simulink model "Main_model"  (R2021b)
settings: Solver=ode23t  StartTime=0.0  StopTime=sim_t_end  RelTol=1e-3
undefined symbols (not defined in the file): ambient_co2, ambient_pressure, ambient_rh, ambient_temp, battery, battery_heat_gen_scale, battery_mass, battery_thermal_mass, cab_air_v_dot, cabin_heater_cmd, cabin_heater_max_power, case_cold_plate_mass, case_cold_plate_thermal_mass, chiller_baffles_n, chiller_tube_length, chiller_tubes_n_rows, compressor_max_m_dot, compressor_ref_m_dot, condenser_air_min_flow_area, condenser_tube_width, const_current, coolant_channel_length, coolant_initial_T, coolant_m_dot, coolant_pipe_cross_sec_area, evaporator_air_cross_sec_area, evaporator_air_min_flow_area, evaporator_tube_width, motor_mc_heat_fraction, n_parallel, power_fraction_rear, ptc_heater_max_power, ptc_heater_thermal_mass, rad_air_v_dot, radiator_air_cross_sec_area, radiator_air_min_flow_area, radiator_tube_width, ref_m_dot, ref_pipe_dia, refrigerant_initial_void_fraction, refrigerant_pipe_cross_sec_area, T_bat_active_cool, T_bat_active_heat, T_bat_passive_cool, T_bat_passive_heat, T_battery_init, T_battery_nom, T_cabin_init, T_cabin_setpoint, T_dcdc_nom, T_DT_high, T_DT_passive_cool, T_DT_whr_active, T_front_gb_nom, T_front_mc_nom, T_front_motor_nom, T_rear_gb_nom, T_rear_mc_nom, T_rear_motor_nom, three_w_valve_max_open_area_factor ... (+3)
libraries: fl_lib x448, nesl_utility x328, SimscapeFluids_lib x134, slpidlib x15, ee_lib x9, simulink x8, LiBatteryElements_lib x4, SignalEditorBlockLib x1
(part 10 of 24)

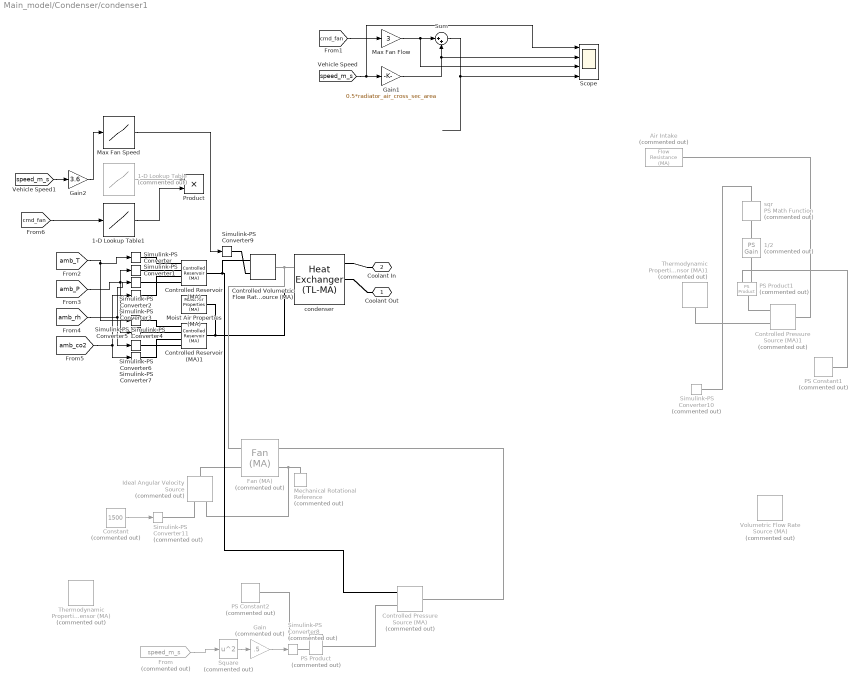
== system Main_model/Condenser/condenser1 ==
  1-D Lookup Table : Lookup_n-D  Commented=on  NumberOfTableDimensions=1  BreakpointsForDimension1=[0, 10, 30, 70, 90,125,161, 180]  Table=[.4462, .4608, .5252, .7346, .8683, 1.2050, 1.5558, 2.15]  InternalRulePriority=Speed  RndMeth=Simplest  InputSameDT=on
  1-D Lookup Table1 : Lookup_n-D  NumberOfTableDimensions=1  BreakpointsForDimension1=[0.5, .75, 1]  Table=[1, 1.15, 1.3]  InternalRulePriority=Speed  RndMeth=Simplest  InputSameDT=on
  1/2 : fl_lib/Physical Signals/Functions/PS Gain  Commented=on  gain=0.5
  Air Intake : fl_lib/Moist Air/Elements/Flow Resistance (MA)  Commented=on  delta_p_nominal=5e-4 MPa  mdot_nominal=1 kg/s  rho_nominal=1.2 kg/m^3  area=.06 m^2  laminar_fraction=1e-3
      settings: SourceProductBaseCode=SS
  Constant : Constant  Commented=on  Value=1500
  Controlled Volumetric Flow Rate Source (MA) : fl_lib/Moist Air/Sources/Controlled Volumetric Flow Rate Source (MA)  power_spec=foundation.enum.power_spec.none  volumetric_flow_conditions=foundation.enum.volumetric_flow_conditions.standard  p_std=0.101325 MPa  T_std=ambient_temp K  RH_std=ambient_rh  area_A=radiator_air_cross_sec_area m^2  area_B=radiator_air_cross_sec_area m^2
      settings: SourceProductBaseCode=SS  InternalSimscapePortConfiguration="{\"Bottom\":[],\"Left\":[{\"id\":\"A\",\"label\":\"A\",\"type\":\"foundation.moist_air.moist_air\"},{\"id\":\"V\",\"label\":\"V\",\"type\":\"input\"}],\"Right\":[{\"id\":\"B\",\"label\":\"B\",\"type\":\"foundation.moist_air.moist_air\"}],\"Top\":[]}"
  Controlled Pressure Source (MA) : fl_lib/Moist Air/Sources/Controlled Pressure Source (MA)  Commented=on  power_spec=foundation.enum.power_spec.none  area_A=0.5*radiator_air_cross_sec_area m^2  area_B=0.5*radiator_air_cross_sec_area m^2
      settings: SourceProductBaseCode=SS  InternalSimscapePortConfiguration="{\"Bottom\":[],\"Left\":[{\"id\":\"A\",\"label\":\"A\",\"type\":\"foundation.moist_air.moist_air\"},{\"id\":\"P\",\"label\":\"P\",\"type\":\"input\"}],\"Right\":[{\"id\":\"B\",\"label\":\"B\",\"type\":\"foundation.moist_air.moist_air\"}],\"Top\":[]}"
  Controlled Pressure Source (MA)1 : fl_lib/Moist Air/Sources/Controlled Pressure Source (MA)  Commented=on  power_spec=foundation.enum.power_spec.isentropic  area_A=.06 m^2  area_B=.06 m^2
      settings: SourceProductBaseCode=SS  InternalSimscapePortConfiguration="{\"Bottom\":[],\"Left\":[{\"id\":\"A\",\"label\":\"A\",\"type\":\"foundation.moist_air.moist_air\"},{\"id\":\"P\",\"label\":\"P\",\"type\":\"input\"}],\"Right\":[{\"id\":\"B\",\"label\":\"B\",\"type\":\"foundation.moist_air.moist_air\"}],\"Top\":[]}"
  Controlled Reservoir (MA) : fl_lib/Moist Air/Elements/Controlled Reservoir (MA)  moisture_spec=foundation.enum.moisture_spec.relative_humidity  trace_gas_spec=foundation.enum.trace_gas_spec.mole_fraction  RH_ws=1  area_A=radiator_air_cross_sec_area m^2  input_error_spec=foundation.enum.input_range_error.warn
      settings: SourceProductBaseCode=SS  InternalSimscapePortConfiguration="{\"Bottom\":[],\"Left\":[{\"id\":\"A\",\"label\":\"A\",\"type\":\"foundation.moist_air.moist_air\"}],\"Right\":[{\"id\":\"T\",\"label\":\"T\",\"type\":\"input\"},{\"id\":\"P\",\"label\":\"P\",\"type\":\"input\"},{\"id\":\"W\",\"label\":\"W\",\"type\":\"input\"},{\"id\":\"G\",\"label\":\"G\",\"type\":\"input\"}],\"Top\":[]}"
  Controlled Reservoir (MA)1 : fl_lib/Moist Air/Elements/Controlled Reservoir (MA)  moisture_spec=foundation.enum.moisture_spec.relative_humidity  trace_gas_spec=foundation.enum.trace_gas_spec.mole_fraction  RH_ws=1  area_A=radiator_air_cross_sec_area m^2  input_error_spec=foundation.enum.input_range_error.warn
      settings: SourceProductBaseCode=SS  InternalSimscapePortConfiguration="{\"Bottom\":[],\"Left\":[{\"id\":\"A\",\"label\":\"A\",\"type\":\"foundation.moist_air.moist_air\"}],\"Right\":[{\"id\":\"T\",\"label\":\"T\",\"type\":\"input\"},{\"id\":\"P\",\"label\":\"P\",\"type\":\"input\"},{\"id\":\"W\",\"label\":\"W\",\"type\":\"input\"},{\"id\":\"G\",\"label\":\"G\",\"type\":\"input\"}],\"Top\":[]}"
  Fan (MA) : SimscapeFluids_lib/Moist Air/Turbomachinery/Fan (MA)  Commented=on  fan_parameterization=fluids.moist_air.turbomachinery.enum.FanParameterization.Nominal  mechanical_power_spec=fluids.moist_air.turbomachinery.enum.FanMechanicalPowerSpec.Power  flow_rate_nominal=1.5 m^3/s  pressure_nominal=300 Pa  eta_nominal=.7  power_nominal=200 W  pressure_max=400 Pa  flow_rate_max=3 m^3/s  omega_ref_nominal=1200 rpm  flow_rate_1D_TLU=[.0278, .0556, .0833, .111, .139, .167] m^3/s  pressure_1D_TLU=[6410, 6375, 6018, 5366, 4501, 3609] Pa  eta_1D_TLU=[.257, .394, .453, .47, .459, .415]  power_1D_TLU=[693, 900, 1107, 1267, 1363, 1452] W  omega_ref_1D=3000 rpm  rho_ref_1D=1.2 kg/m^3  omega_dp_TLU=[2400; 3000; 3600] rpm  flow_rate_dp_TLU=[.0278, .0556, .0833, .111, .139, .167] m^3/s  pressure_dp_TLU=[4111, 4010, 3551, 2881, 2167, 1453; 6410, 6375, 6018, 5366, 4501, 3609; 9217, 9285, 9022, 8428, 7552, 6482] Pa  eta_dp_TLU=[.3, .434, .468, .459, .4, .3; .257, .394, .453, .47, .459, .415; .225, .359, .434, .461, .47, .459]  power_dp_TLU=[381, 514, 632, 697, 753, 809; 693, 900, 1107, 1267, 1363, 1452; 1139, 1438, 1732, 2029, 2233, 2358] W  rho_ref_dp=1.2 kg/m^3  omega_q_TLU=[2990; 3450; 3867] rpm  pressure_q_TLU=[31, 62, 93, 124] Pa  flow_rate_q_TLU=[.802, .759, .703, .611; .936, .902, .862, .81; 1.056, 1.027, .994, .956] m^3/s  eta_q_TLU=[.088, .162, .22, .261; .068, .128, .18, .222; .055, .105, .148, .188]  power_q_TLU=[283, 290, 297, 290; 427, 437, 445, 452; 595, 606, 625, 631] W  rho_ref_q=1.2 kg/m^3  diameter_ratio=1  mech_orientation=fluids.moist_air.turbomachinery.enum.FanMechanicalOrientation.Positive  area_A=0.5*radiator_air_cross_sec_area m^2  area_B=0.5*radiator_air_cross_sec_area m^2
      settings: SourceProductBaseCode=SH  InternalSimscapePortConfiguration="{\"Bottom\":[],\"Left\":[{\"id\":\"A\",\"label\":\"A\",\"type\":\"foundation.moist_air.moist_air\"},{\"id\":\"C\",\"label\":\"C\",\"type\":\"foundation.mechanical.rotational.rotational\"}],\"Right\":[{\"id\":\"B\",\"label\":\"B\",\"type\":\"foundation.moist_air.moist_air\"},{\"id\":\"R\",\"label\":\"R\",\"type\":\"foundation.mechanical.rotational.rotational\"}],\"Top\":[]}"
  From : From  Commented=on  GotoTag=speed_m_s  TagVisibility=global
  Gain : Gain  Commented=on  Gain=.5
  Gain1 : Gain  Gain=0.5*radiator_air_cross_sec_area
  Gain2 : Gain  Gain=3.6
  Ideal Angular Velocity Source : fl_lib/Mechanical/Mechanical Sources/Ideal Angular Velocity Source  Commented=on
  Max Fan Flow : Gain  Gain=3
  Max Fan Speed : Lookup_n-D  NumberOfTableDimensions=1  BreakpointsForDimension1=[0, 10, 30, 70, 90,125,161, 180]  Table=[.76, .78, .81, 1.0, 1.1, 1.36, 1.65, 2.21]  InternalRulePriority=Speed  RndMeth=Simplest  InputSameDT=on
  Mechanical Rotational Reference : fl_lib/Mechanical/Rotational Elements/Mechanical Rotational Reference  Commented=on
  Moist Air Properties (MA) : fl_lib/Moist Air/Utilities/Moist Air Properties (MA)  R_a=287.047 J/(K*kg)  T_TLU=[-56.55, -50 : 10 : -10, -5 : 1 : 5, 10 : 10 : 350]' degC  h_a_TLU=[342.416126230579; 349.005511058471; 359.063577249119; 369.119948684177; 379.175469465129; 389.230944678417; 394.258910928084; 395.264534937366; 396.27017101329; 397.275819932805; 398.281482472874; 399.287159410541; 400.292851523015; 401.298559587728; 402.304284382408; 403.310026685143; 404.315787274435; 409.34489180313; 419.404921755863; 429.468036401264; 439.535033154839; 449.606720928652; 459.683919949603; 469.767460521911; 479.858181001348; 489.956925196484; 500.064539372946; 510.181869006204; 520.309755403634; 530.449032296018; 540.60052248087; 550.765034584465; 560.943359995745; 571.136270013102; 581.344513234296; 591.568813210327; 601.809866375885; 612.068340261954; 622.344871990218; 632.640067043998; 642.95449830646; 653.288705353699; 663.643193987949; 674.018435994423; 684.414869104228; 694.832897145098; 705.272890361557; 715.735185886199; 726.220088344236; 736.727870574087; 747.258774447567; 757.813011774199] kJ/kg  mu_a_TLU=[14.2568883320012; 14.6140127728333; 15.1517277055779; 15.6806860159119; 16.2012351072083; 16.7137043125028; 16.9670071730589; 17.017438062815; 17.0677930842452; 17.1180725309876; 17.1682766951315; 17.2184058672268; 17.2684603362935; 17.3184403898301; 17.3683463138234; 17.4181783927569; 17.4679369096204; 17.7156358640698; 18.2056751785154; 18.68879035749; 19.1652344664982; 19.6352478927873; 20.099059103658; 20.5568853601578; 21.0089333871663; 21.4554000014051; 21.8964726992323; 22.3323302062775; 22.7631429910631; 23.1890737447833; 23.6102778293792; 24.0269036959922; 24.4390932757886; 24.8469823450548; 25.2507008663546; 25.6503733074314; 26.0461189394339; 26.4380521159325; 26.8262825340948; 27.2109154792923; 27.5920520543128; 27.969789394274; 28.3442208682439; 28.7154362685068; 29.0835219883356; 29.4485611890712; 29.8106339572472; 30.1698174524429; 30.5261860464955; 30.8798114546565; 31.2307628592324; 31.5791070262086] s*uPa  k_a_TLU=[19.8808489374933; 20.4162454629695; 21.2248743590758; 22.0232452890903; 22.8117314495857; 23.5906913619588; 23.9767075412237; 24.053639990175; 24.1304826682191; 24.2072359051629; 24.2839000294007; 24.3604753679152; 24.4369622462801; 24.5133609886625; 24.5896719178249; 24.6658953551279; 24.7420316205333; 25.1214164701832; 25.8738283029331; 26.6180150229276; 27.3542674377332; 28.0828634735341; 28.8040686837224; 29.5181367785657; 30.2253101618423; 30.9258204644224; 31.6198890677835; 32.3077276126633; 32.9895384896798; 33.6655153099498; 34.33584335461; 35.0007000027879; 35.6602551380254; 36.3146715334901; 36.9641052165342; 37.6087058133173; 38.248616874307; 38.8839761815308; 39.5149160384798; 40.1415635435708; 40.7640408480637; 41.3824653993118; 41.9969501701893; 42.6076038755117; 43.2145311762238; 43.8178328720941; 44.4176060836121; 45.013944423749; 45.6069381602018; 46.1966743687041; 46.783237077953; 47.3667074066625] mW/(K*m)  p_min=1 kPa  p_max=inf MPa  T_min=-56.55 degC  T_max=350 degC  p_atm=ambient_pressure MPa  T_atm=ambient_temp K  R_w=461.523 J/(K*kg)  p_ws_TLU=[1.71168953425982e-06; 3.93770601979424e-06; 1.28411717710344e-05; 3.80051394873809e-05; .00010323902900209; .000259873810798063; .000401741022116384; .000437454836117844; .000476040820618202; .000517704666185737; .000562664883741207; .000611212677444345; .000657088049117899; .000705987905898279; .000758082381149132; .000813549384183233; .000872574861129522; .00122818386934022; .0023392147667769; .00424668834054807; .00738442748706953; .0123512704340234; .0199458019246787; .0312006356960619; .0474147199263783; .0701823607447713; .10141797792131; .143375967241115; .198665399739302; .270259606559999; .361500961984849; .476101381081492; .618139196722055; .792053183687694; 1.0026345688121; 1.25501792086105; 1.55467186826983; 1.90739066433297; 2.31928772772542; 2.79679245576864; 3.34665187151016; 3.97593907083533; 4.69207105435535; 5.5028394740883; 6.41645928168037; 7.4416425436169; 8.58770832955728; 9.86474556030261; 11.2838558865497; 12.8575218898034; 14.6001810568052; 16.5291642526045] MPa  h_w_vap_TLU=[2836.88241275372; 2837.81392500514; 2838.63937175807; 2838.7309929628; 2838.06905313927; 2836.62597341095; 2835.60023952573; 2835.37006381376; 2835.13143158077; 2834.88429145066; 2834.62859062897; 2500.93420564316; 2498.55329907119; 2496.17495082036; 2493.79885912205; 2491.42474723191; 2489.05236104642; 2477.20875029194; 2453.54955988604; 2429.83856603313; 2406.00136954922; 2381.97406342174; 2357.69101156389; 2333.08088387814; 2308.06565480412; 2282.56034405021; 2256.47287422313; 2229.70428017508; 2202.14968030993; 2173.69998896199; 2144.24368406447; 2113.66758247452; 2081.85585110571; 2048.68725710494; 2014.03141249899; 1977.7449923284; 1939.66849592886; 1899.62342931686; 1857.40930169838; 1812.79975416601; 1765.53721731251; 1715.32525772152; 1661.81700477787; 1604.59703745016; 1543.1534616334; 1476.83692476464; 1404.80240352424; 1325.92091736114; 1238.61667822208; 1140.5102987018; 1027.62017777647; 892.733785613825] kJ/kg  h_w_TLU=[2396.55944251649; 2408.68643343608; 2427.1988031141; 2445.702165897; 2464.18429108356; 2482.62529466839; 2491.82135326629; 2493.6580151792; 2495.49372578218; 2497.32843835745; 2499.16210446923; 2500.99462758899; 2502.83092214066; 2504.6665223621; 2506.50140563013; 2508.335548891; 2510.16892865793; 2519.32352241995; 2537.56068088674; 2555.67742615292; 2573.6403223998; 2591.4109179101; 2608.9455037701; 2626.19492016262; 2643.10444358428; 2659.61377634497; 2675.58278696023; 2696.1846256545; 2716.49989553741; 2736.6235210957; 2756.61216047011; 2776.50561773853; 2796.33378922508; 2816.11979583049; 2835.88181423877; 2855.63430574511; 2875.38889327595; 2895.15500577172; 2914.94035964689; 2934.75132290228; 2954.59319330244; 2974.47041285505; 2994.38673458964; 3014.34535328009; 3034.34900867103; 3054.40006755764; 3074.50058946898; 3094.65237953784; 3114.85703128106; 3135.11596137801; 3155.43043805905; 3175.80160435813] kJ/kg  mu_w_TLU=[6.81365662228272; 7.04953750742707; 7.40970098298307; 7.76991278093907; 8.13017290129507; 8.49048134405107; 8.67065368632907; 8.70668960445667; 8.74272600580827; 8.77876289038387; 8.81480025818347; 8.85083810920707; 8.88687644345467; 8.92291526092627; 8.95895456162187; 8.99499434554147; 9.03103461268507; 9.21124319676307; 9.57169660671907; 9.93219833907507; 10.2927483938311; 10.6533467709871; 11.0139934705431; 11.3746884924991; 11.7354318368551; 12.0962235036111; 12.4570634927671; 12.8179518043231; 13.1788884382791; 13.5398733946351; 13.9009066733911; 14.2619882745471; 14.6231181981031; 14.9842964440591; 15.3455230124151; 15.7067979031711; 16.0681211163271; 16.4294926518831; 16.7909125098391; 17.1523806901951; 17.5138971929511; 17.8754620181071; 18.2370751656631; 18.5987366356191; 18.9604464279751; 19.3222045427311; 19.6840109798871; 20.0458657394431; 20.4077688213991; 20.7697202257551; 21.1317199525111; 21.4937680016671] s*uPa  k_w_TLU=[11.46288215976; 11.941997488935; 12.676358586935; 13.414208884935; 14.155548382935; 14.900377080935; 15.274099879935; 15.348949115735; 15.423833243535; 15.498752263335; 15.573706175135; 15.648694978935; 15.723718674735; 15.798777262535; 15.873870742335; 15.948999114135; 16.024162377935; 16.400502076935; 17.155798374935; 17.914583872935; 18.676858570935; 19.442622468935; 20.211875566935; 20.984617864935; 21.760849362935; 22.540570060935; 23.323779958935; 24.110479056935; 24.900667354935; 25.694344852935; 26.491511550935; 27.292167448935; 28.096312546935; 28.903946844935; 29.715070342935; 30.529683040935; 31.347784938935; 32.169376036935; 32.994456334935; 33.823025832935; 34.655084530935; 35.490632428935; 36.329669526935; 37.172195824935; 38.018211322935; 38.867716020935; 39.720709918935; 40.577193016935; 41.437165314935; 42.300626812935; 43.167577510935; 44.038017408935] mW/(K*m)  D_w=25 mm^2/s  trace_gas_model=foundation.enum.trace_gas_model.none  R_g=188.923 J/(K*kg)  h_g_TLU=[439.555216260064; 444.670268200251; 452.538618847003; 460.487124258496; 468.522588768941; 476.649415958793; 480.74798538725; 481.57054318762; 482.394052398751; 483.218514288831; 484.043930029015; 484.870300696555; 485.697627277859; 486.525910671489; 487.355151691079; 488.185351068185; 489.016509455051; 493.186704139431; 501.599194953048; 510.107689961685; 518.711611080182; 527.410026793075; 536.201764778798; 545.085474203452; 554.059675505208; 563.122805485367; 572.27325096919; 581.509373027928; 590.829525105886; 600.232066705818; 609.715373581392; 619.277845178105; 628.917909922924; 638.634028838794; 648.424697859328; 658.288449140109; 668.223851601449; 678.229510889093; 688.304068901113; 698.44620299875; 708.654624994591; 718.928079991818; 729.265345132425; 739.665228299475; 750.126566808087; 760.648226111439; 771.229098541268; 781.868102096908; 792.564179292476; 803.316296068366; 814.123440770426; 824.984623198037] kJ/kg  mu_g_TLU=[10.8921054191698; 11.2215357085649; 11.7233300740382; 12.2234238147811; 12.7215124453467; 13.2173328890673; 13.4643203184773; 13.5136406274989; 13.562934752385; 13.6122025024997; 13.6614436900741; 13.7106581301692; 13.7598456406398; 13.8090060420983; 13.8581391578796; 13.9072448140062; 13.9563228391538; 14.2012926853717; 14.6890687376044; 15.1738428124161; 15.6554929043332; 16.1339159800463; 16.6090257998657; 17.0807510097148; 17.5490334645512; 18.0138267508952; 18.4750948814453; 18.9328111390399; 19.3869570507278; 19.8375214755778; 20.2844997922255; 20.7278931741254; 21.1677079421287; 21.6039549853963; 22.036649242835; 22.4658092382469; 22.8914566632375; 23.3136160026627; 23.7323141980278; 24.1475803447965; 24.5594454200432; 24.9679420372927; 25.3731042257492; 25.774967231431; 26.1735673380029; 26.5689417053362; 26.9611282240413; 27.350165384404; 27.73609215832; 28.118947892972; 28.4987722151178; 28.8756049449796] s*uPa  k_g_TLU=[10.489430678843; 10.9507672150864; 11.666197960308; 12.392559739764; 13.1299519771612; 13.8778409888416; 14.2554325416312; 14.3312274189707; 14.4071122346908; 14.4830860227061; 14.5591478179508; 14.6352966574703; 14.7115315815553; 14.787851634907; 14.8642558678259; 14.9407433374142; 15.0173131087819; 15.401364480906; 16.1751373988038; 16.9558134611595; 17.7432208682398; 18.5366976599676; 19.3360988502003; 20.1412225692689; 20.9517507672929; 21.7672310558863; 22.5871115634685; 23.4107980865695; 24.2377021890869; 25.0672663781241; 25.8989689893876; 26.732318357514; 27.5668446164644; 28.4020933015927; 29.2376215872816; 30.0729965057542; 30.9077942826816; 31.7416001931033; 32.5740086297993; 33.4046232539953; 34.2330571812868; 35.0589331874899; 35.8818839295189; 36.701552179391; 37.5175910702657; 38.3296643536716; 39.1374466671854; 39.9406238119064; 40.7388930391313; 41.5319633456945; 42.3195557774861; 43.1014037407076] mW/(K*m)  D_g=16 mm^2/s
      settings: SourceProductBaseCode=SS
  PS Constant1 : fl_lib/Physical Signals/Sources/PS Constant  Commented=on  constant=1.2 kg/m^3
  PS Constant2 : fl_lib/Physical Signals/Sources/PS Constant  Commented=on  constant=1.2 kg/m^3
  PS Product : fl_lib/Physical Signals/Functions/PS Product  Commented=on
  PS Product1 : fl_lib/Physical Signals/Functions/PS Product  Commented=on
  Product : Product
  Scope : Scope  NumInputPorts=4
  Simulink-PS Converter : nesl_utility/Simulink-PS Converter  PhysicalDomain=network_engine_domain  SubClassName=ps_input  LeftPortType=input  RightPortType=output  PseudoPeriodic=off  Frequencies=[]  NoiseDistribution=none  NoiseParameters=[]  Unit=K  AffineConversion=off  FilteringAndDerivatives=provide  SimscapeFilterOrder=1  InputFilterTimeConstant=0.001  UdotUserProvided=0
      settings: SourceProductBaseCode=PW,SS
  Simulink-PS Converter1 : nesl_utility/Simulink-PS Converter  PhysicalDomain=network_engine_domain  SubClassName=ps_input  LeftPortType=input  RightPortType=output  PseudoPeriodic=off  Frequencies=[]  NoiseDistribution=none  NoiseParameters=[]  Unit=MPa  AffineConversion=off  FilteringAndDerivatives=provide  SimscapeFilterOrder=1  InputFilterTimeConstant=0.001  UdotUserProvided=0
      settings: SourceProductBaseCode=PW,SS
  Simulink-PS Converter10 : nesl_utility/Simulink-PS Converter  Commented=on  PhysicalDomain=network_engine_domain  SubClassName=ps_input  LeftPortType=input  RightPortType=output  PseudoPeriodic=off  Frequencies=[]  NoiseDistribution=none  NoiseParameters=[]  Unit=m/s  AffineConversion=off  FilteringAndDerivatives=provide  SimscapeFilterOrder=1  InputFilterTimeConstant=0.001  UdotUserProvided=0
      settings: SourceProductBaseCode=PW,SS
  Simulink-PS Converter11 : nesl_utility/Simulink-PS Converter  Commented=on  PhysicalDomain=network_engine_domain  SubClassName=ps_input  LeftPortType=input  RightPortType=output  PseudoPeriodic=off  Frequencies=[]  NoiseDistribution=none  NoiseParameters=[]  Unit=rpm  AffineConversion=off  FilteringAndDerivatives=provide  SimscapeFilterOrder=1  InputFilterTimeConstant=0.001  UdotUserProvided=0
      settings: SourceProductBaseCode=PW,SS
  Simulink-PS Converter{2..3,6..7} (4 alike) : nesl_utility/Simulink-PS Converter  PhysicalDomain=network_engine_domain  SubClassName=ps_input  LeftPortType=input  RightPortType=output  PseudoPeriodic=off  Frequencies=[]  NoiseDistribution=none  NoiseParameters=[]  Unit=1  AffineConversion=off  FilteringAndDerivatives=provide  SimscapeFilterOrder=1  InputFilterTimeConstant=0.001  UdotUserProvided=0
      settings: SourceProductBaseCode=PW,SS
  Simulink-PS Converter4 : nesl_utility/Simulink-PS Converter  PhysicalDomain=network_engine_domain  SubClassName=ps_input  LeftPortType=input  RightPortType=output  PseudoPeriodic=off  Frequencies=[]  NoiseDistribution=none  NoiseParameters=[]  Unit=K  AffineConversion=off  FilteringAndDerivatives=provide  SimscapeFilterOrder=1  InputFilterTimeConstant=0.001  UdotUserProvided=0
      settings: SourceProductBaseCode=PW,SS
  Simulink-PS Converter5 : nesl_utility/Simulink-PS Converter  PhysicalDomain=network_engine_domain  SubClassName=ps_input  LeftPortType=input  RightPortType=output  PseudoPeriodic=off  Frequencies=[]  NoiseDistribution=none  NoiseParameters=[]  Unit=MPa  AffineConversion=off  FilteringAndDerivatives=provide  SimscapeFilterOrder=1  InputFilterTimeConstant=0.001  UdotUserProvided=0
      settings: SourceProductBaseCode=PW,SS
  Simulink-PS Converter8 : nesl_utility/Simulink-PS Converter  Commented=on  PhysicalDomain=network_engine_domain  SubClassName=ps_input  LeftPortType=input  RightPortType=output  PseudoPeriodic=off  Frequencies=[]  NoiseDistribution=none  NoiseParameters=[]  Unit=m^2/s^2  AffineConversion=off  FilteringAndDerivatives=provide  SimscapeFilterOrder=1  InputFilterTimeConstant=0.001  UdotUserProvided=0
      settings: SourceProductBaseCode=PW,SS
  Simulink-PS Converter9 : nesl_utility/Simulink-PS Converter  PhysicalDomain=network_engine_domain  SubClassName=ps_input  LeftPortType=input  RightPortType=output  PseudoPeriodic=off  Frequencies=[]  NoiseDistribution=none  NoiseParameters=[]  Unit=m^3/s  AffineConversion=off  FilteringAndDerivatives=provide  SimscapeFilterOrder=1  InputFilterTimeConstant=0.001  UdotUserProvided=0
      settings: SourceProductBaseCode=PW,SS
  Square : Math  Commented=on  Operator=square  SaturateOnIntegerOverflow=on
  Sum : Sum  Inputs=|++
  Thermodynamic Properties Sensor (MA) : fl_lib/Moist Air/Sensors/Thermodynamic Properties Sensor (MA)  Commented=on  measurement_mass_spec=foundation.enum.measurement_mass_spec.mixture
      settings: SourceProductBaseCode=SS  InternalSimscapePortConfiguration="{\"Bottom\":[],\"Left\":[{\"id\":\"A\",\"label\":\"A\",\"type\":\"foundation.moist_air.moist_air\"}],\"Right\":[{\"id\":\"H\",\"label\":\"h\",\"type\":\"output\"},{\"id\":\"RHO\",\"label\":\"rho\",\"type\":\"output\"},{\"id\":\"CP\",\"label\":\"cp\",\"type\":\"output\"},{\"id\":\"S\",\"label\":\"s\",\"type\":\"output\"}],\"Top\":[]}"
  Thermodynamic Properties Sensor (MA)1 : fl_lib/Moist Air/Sensors/Thermodynamic Properties Sensor (MA)  Commented=on  measurement_mass_spec=foundation.enum.measurement_mass_spec.mixture
      settings: SourceProductBaseCode=SS  InternalSimscapePortConfiguration="{\"Bottom\":[],\"Left\":[{\"id\":\"A\",\"label\":\"A\",\"type\":\"foundation.moist_air.moist_air\"}],\"Right\":[{\"id\":\"H\",\"label\":\"h\",\"type\":\"output\"},{\"id\":\"RHO\",\"label\":\"rho\",\"type\":\"output\"},{\"id\":\"CP\",\"label\":\"cp\",\"type\":\"output\"},{\"id\":\"S\",\"label\":\"s\",\"type\":\"output\"}],\"Top\":[]}"
  Volumetric Flow Rate Source (MA) : fl_lib/Moist Air/Sources/Volumetric Flow Rate Source (MA)  Commented=on  power_spec=foundation.enum.power_spec.none  volumetric_flow=1 m^3/s  volumetric_flow_conditions=foundation.enum.volumetric_flow_conditions.standard  p_std=0.101325 MPa  T_std=ambient_temp K  RH_std=ambient_rh  area_A=.06 m^2  area_B=.06 m^2
      settings: SourceProductBaseCode=SS  InternalSimscapePortConfiguration="{\"Bottom\":[],\"Left\":[{\"id\":\"A\",\"label\":\"A\",\"type\":\"foundation.moist_air.moist_air\"}],\"Right\":[{\"id\":\"B\",\"label\":\"B\",\"type\":\"foundation.moist_air.moist_air\"}],\"Top\":[]}"
  condenser : SimscapeFluids_lib/Fluid Network Interfaces/Heat Exchangers/Heat Exchanger (TL-MA)  flow_arrangement=fluids.interfaces.heat_exchangers.enum.FlowArrangementTLMA.Cross  cross_flow_arrangement=fluids.interfaces.heat_exchangers.enum.CrossFlowArrangementTLMA.UnmixedMixed  R_wall=radiator_wall_thermal_resistance K/W  area_A1=coolant_pipe_cross_sec_area m^2  area_B1=coolant_pipe_cross_sec_area m^2  area_A2=radiator_air_cross_sec_area m^2  area_B2=radiator_air_cross_sec_area m^2  flow_geometry_TL=fluids.interfaces.heat_exchangers.enum.FlowGeometryTL.InsideTubes  tube_num_TL=radiator_n_tubes  tube_length_TL=radiator_tube_length m  tube_cross_section_TL=fluids.interfaces.heat_exchangers.enum.TubeCrossSection.Rectangular  tube_diameter_TL=0.05 m  tube_width_TL=radiator_tube_width m  tube_height_TL=radiator_tube_height m  tube_inner_diameter_TL=0.05 m  tube_outer_diameter_TL=0.1 m  tube_flow_area_TL=0.002 m^2  tube_wetted_perimeter_TL=0.15 m  tube_heat_perimeter_TL=0.15 m  tube_pressure_loss_spec_TL=fluids.interfaces.heat_exchangers.enum.TubePressureLossSpec.Haaland  tube_loss_coeff_TL=10  tube_length_add_TL=radiator_tube_eqv_resistance_length m  tube_roughness_pressure_TL=15e-6 m  tube_Re_lam_pressure_TL=2000  tube_Re_tur_pressure_TL=4000  tube_shape_factor_generic_TL=64  tube_heat_coeff_spec_TL=fluids.interfaces.heat_exchangers.enum.TubeHeatCoeffSpec.Gneilinski  tube_colburn_coeff_TL=rad_coolant_side_coef  tube_roughness_heat_TL=15e-6 m  tube_Re_lam_heat_TL=2000  tube_Re_tur_heat_TL=4000  tube_Nu_lam_generic_TL=3.66  bank_arrangement_TL=fluids.interfaces.heat_exchangers.enum.BankArrangement.Inline  bank_num_rows_TL=5  bank_tubes_per_row_TL=5  bank_width_TL=1 m  bank_tube_diameter_TL=0.05 m  bank_longitudinal_pitch_TL=0.15 m  bank_transverse_pitch_TL=0.15 m  bank_pressure_loss_spec_TL=fluids.interfaces.heat_exchangers.enum.BankPressureLossSpec.Martin  bank_euler_TL=10  bank_heat_coeff_spec_TL=fluids.interfaces.heat_exchangers.enum.BankHeatCoeffSpec.Martin  bank_colburn_coeff_TL=[.27, .63, .36]  generic_flow_area_TL=0.01 m^2  generic_heat_area_TL=2 m^2  generic_volume_TL=0.05 m^3  generic_loss_coeff_TL=10  generic_colburn_coeff_TL=[.023, .8, .33]  fouling_factor_TL=0 K*m^2/kW  fin_area_TL=0 m^2  fin_efficiency_TL=0  p_init_TL=coolant_initial_P MPa  T_init_TL=coolant_initial_T K  flow_geometry_MA=fluids.interfaces.heat_exchangers.enum.FlowGeometryMA.Generic  tube_num_MA=25  tube_length_MA=1 m  tube_cross_section_MA=fluids.interfaces.heat_exchangers.enum.TubeCrossSection.Circular  tube_diameter_MA=0.05 m  tube_width_MA=0.05 m  tube_height_MA=0.05 m  tube_inner_diameter_MA=0.05 m  tube_outer_diameter_MA=0.1 m  tube_flow_area_MA=0.002 m^2  tube_wetted_perimeter_MA=0.15 m  tube_heat_perimeter_MA=0.15 m  tube_pressure_loss_spec_MA=fluids.interfaces.heat_exchangers.enum.TubePressureLossSpec.Haaland  tube_loss_coeff_MA=10  tube_length_add_MA=0.1 m  tube_roughness_pressure_MA=15e-6 m  tube_Re_lam_pressure_MA=2000  tube_Re_tur_pressure_MA=4000  tube_shape_factor_generic_MA=64  tube_heat_coeff_spec_MA=fluids.interfaces.heat_exchangers.enum.TubeHeatCoeffSpec.Gneilinski  tube_colburn_coeff_MA=[.023, .8, .33]  tube_roughness_heat_MA=15e-6 m  tube_Re_lam_heat_MA=2000  tube_Re_tur_heat_MA=4000  tube_Nu_lam_generic_MA=3.66  bank_arrangement_MA=fluids.interfaces.heat_exchangers.enum.BankArrangement.Inline  bank_num_rows_MA=1  bank_tubes_per_row_MA=radiator_n_tubes  bank_width_MA=radiator_tube_length m  bank_tube_diameter_MA=radiator_tube_height m  bank_longitudinal_pitch_MA=radiator_tube_pitch m  bank_transverse_pitch_MA=radiator_tube_pitch m  bank_pressure_loss_spec_MA=fluids.interfaces.heat_exchangers.enum.BankPressureLossSpec.Martin  bank_euler_MA=10  bank_heat_coeff_spec_MA=fluids.interfaces.heat_exchangers.enum.BankHeatCoeffSpec.Colburn  bank_colburn_coeff_MA=rad_air_side_coef  generic_flow_area_MA=radiator_air_min_flow_area m^2  generic_heat_area_MA=radiator_ht_surf_area_without_fins m^2  generic_volume_MA=radiator_air_min_flow_area*radiator_tube_width m^3  generic_loss_coeff_MA=4  generic_colburn_coeff_MA=rad_air_side_coef  fouling_factor_MA=0 K*m^2/kW  fin_area_MA=radiator_fin_surf_area m^2  fin_efficiency_MA=radiator_air_fin_eff  p_init_MA=ambient_pressure MPa  T_init_MA=ambient_temp K  moisture_spec_MA=foundation.enum.moisture_spec.relative_humidity  RH_init_MA=ambient_rh  x_w_init_MA=0.01  y_w_init_MA=0.01  HR_init_MA=0.01  trace_gas_spec_MA=foundation.enum.trace_gas_spec.mole_fraction  x_g_init_MA=ambient_co2  y_g_init_MA=ambient_co2  RH_ws_MA=1
      settings: SourceProductBaseCode=SH  InternalSimscapePortConfiguration="{\"Bottom\":[],\"Left\":[{\"id\":\"A1\",\"label\":\"A1\",\"type\":\"foundation.thermal_liquid.thermal_liquid\"},{\"id\":\"B1\",\"label\":\"B1\",\"type\":\"foundation.thermal_liquid.thermal_liquid\"}],\"Right\":[{\"id\":\"A2\",\"label\":\"A2\",\"type\":\"foundation.moist_air.moist_air\"},{\"id\":\"B2\",\"label\":\"B2\",\"type\":\"foundation.moist_air.moist_air\"}],\"Top\":[{\"id\":\"W\",\"label\":\"W\",\"type\":\"output\"}]}"
  sqr : fl_lib/Physical Signals/Functions/PS Math Function  Commented=on  fcn_choice=foundation.enum.math_function.square  v=1
      settings: SourceProductBaseCode=SS
  Coolant Out : PMIOPort  Side=Right
  Coolant In : PMIOPort  Port=2  Side=Right
  wires:
  [amb_P] -> Simulink-PS Converter1/1, Simulink-PS Converter5/1
  [amb_co2] -> Simulink-PS Converter3/1, Simulink-PS Converter7/1
  Square/1 -> Gain/1
  From/1 -> Square/1
  Gain/1 -> Simulink-PS Converter8/1
  [amb_rh] -> Simulink-PS Converter2/1, Simulink-PS Converter6/1
  [amb_T] -> Simulink-PS Converter/1, Simulink-PS Converter4/1
  [speed_m_s] -> Gain1/1, Scope/1
  Constant/1 -> Simulink-PS Converter11/1
  [cmd_fan] -> Max Fan Flow/1
  Sum/1 -> Scope/4
  Max Fan Flow/1 -> Scope/3, Sum/1
  Gain1/1 -> Sum/2, Scope/2
  [speed_m_s] -> Gain2/1
  1-D Lookup Table/1 -> Product/1
  [cmd_fan] -> 1-D Lookup Table1/1
  Gain2/1 -> Max Fan Speed/1
  1-D Lookup Table1/1 -> Product/2
  Max Fan Speed/1 -> Simulink-PS Converter9/1
  connections:
  Simulink-PS Converter/RConn1 -- Controlled Reservoir (MA)/RConn1
  Simulink-PS Converter1/RConn1 -- Controlled Reservoir (MA)/RConn2
  Simulink-PS Converter4/RConn1 -- Controlled Reservoir (MA)1/RConn1
  Simulink-PS Converter2/RConn1 -- Controlled Reservoir (MA)/RConn3
  PS Product/RConn1 -- Controlled Pressure Source (MA)/LConn2
  PS Product/LConn2 -- Simulink-PS Converter8/RConn1
  Simulink-PS Converter3/RConn1 -- Controlled Reservoir (MA)/RConn4
  Simulink-PS Converter5/RConn1 -- Controlled Reservoir (MA)1/RConn2
  condenser/LConn1 -- Coolant In/RConn1
  Simulink-PS Converter7/RConn1 -- Controlled Reservoir (MA)1/RConn4
  Simulink-PS Converter6/RConn1 -- Controlled Reservoir (MA)1/RConn3
  condenser/LConn2 -- Coolant Out/RConn1
  1/2/RConn1 -- PS Product1/LConn1
  Simulink-PS Converter10/RConn1 -- sqr/LConn1
  PS Product1/RConn1 -- Controlled Pressure Source (MA)1/LConn2
  sqr/RConn1 -- 1/2/LConn1
  PS Constant1/RConn1 -- PS Product1/LConn2
  Air Intake/LConn1 -- Controlled Pressure Source (MA)1/RConn1
  Thermodynamic Properties Sensor (MA)1/LConn1 -- Controlled Pressure Source (MA)1/LConn1
  Controlled Reservoir (MA)1/LConn1 -- condenser/RConn2 -- Moist Air Properties (MA)/RConn1
  Simulink-PS Converter9/RConn1 -- Controlled Volumetric Flow Rate Source (MA)/LConn2
  Fan (MA)/LConn2 -- Ideal Angular Velocity Source/RConn2 -- Mechanical Rotational Reference/LConn1
  Ideal Angular Velocity Source/LConn1 -- Fan (MA)/RConn2
  Simulink-PS Converter11/RConn1 -- Ideal Angular Velocity Source/RConn1
  PS Constant2/RConn1 -- PS Product/LConn1
  Controlled Reservoir (MA)/LConn1 -- Controlled Volumetric Flow Rate Source (MA)/LConn1 -- Controlled Pressure Source (MA)/LConn1
  Controlled Pressure Source (MA)/RConn1 -- Fan (MA)/LConn1
  Fan (MA)/RConn1 -- condenser/RConn1 -- Controlled Volumetric Flow Rate Source (MA)/RConn1

== system Main_model/HP Control Systems Battery to Chiller WHR /HysBat ==
  In1 : Inport
  Relay1 : Relay  OnSwitchValue=T_bat_passive_cool  OffSwitchValue=T_bat_passive_cool-1  OnOutputValue=T_bat_passive_cool*1.1  OffOutputValue=T_bat_passive_cool*.9
  Relay3 : Relay  OnSwitchValue=T_bat_active_cool  OffSwitchValue=T_bat_active_cool-1  OnOutputValue=T_bat_active_cool*1.1  OffOutputValue=T_bat_active_cool*.9
  Switch : Switch  Criteria=u2 > Threshold  Threshold=T_bat_active_cool-5
  Switch1 : Switch  Criteria=u2 > Threshold  Threshold=T_bat_passive_cool-5
  Out1 : Outport
  wires:
  Relay3/1 -> Switch/1
  Switch/1 -> Out1/1
  Relay1/1 -> Switch1/1
  In1/1 -> Relay1/1, Relay3/1, Switch/2, Switch1/2, Switch1/3
  Switch1/1 -> Switch/3

== system Main_model/HP Control Systems Battery to Chiller WHR /HysDT ==
  In1 : Inport
  Relay2 : Relay  OnSwitchValue=T_DT_passive_cool  OffSwitchValue=T_DT_passive_cool-9  OnOutputValue=T_DT_passive_cool*1.1  OffOutputValue=T_DT_passive_cool*.9
  Relay3 : Relay  OnSwitchValue=T_DT_high  OffSwitchValue=T_DT_high-20  OnOutputValue=T_DT_high*1.1  OffOutputValue=T_DT_high*.9
  Switch : Switch  Criteria=u2 > Threshold  Threshold=T_DT_passive_cool+10
  Out1 : Outport
  wires:
  Relay2/1 -> Switch/3
  Switch/1 -> Out1/1
  Relay3/1 -> Switch/1
  In1/1 -> Relay2/1, Switch/2, Relay3/1

== system Main_model/HP Control Systems Battery to Chiller WHR /TF ==
  In1 : Inport
  Constant : Constant  Value=T_battery_init
  Sum5 : Sum  Inputs=|++
  Sum6 : Sum  Inputs=|-+
  Transfer Fcn15 : TransferFcn  Denominator=[60 1]
  Transfer Fcn16 : TransferFcn  Denominator=[60 1]
  Out1 : Outport
  wires:
  Constant/1 -> Sum6/2, Transfer Fcn16/1
  Sum6/1 -> Sum5/2
  Sum5/1 -> Out1/1
  Transfer Fcn15/1 -> Sum5/1
  Transfer Fcn16/1 -> Sum6/1
  In1/1 -> Transfer Fcn15/1

== system Main_model/HP Control Systems Battery to Chiller WHR /TF1 ==
  In1 : Inport
  Constant : Constant  Value=T_cabin_init
  Sum5 : Sum  Inputs=|++
  Sum6 : Sum  Inputs=|-+
  Transfer Fcn15 : TransferFcn  Denominator=[15 1]
  Transfer Fcn16 : TransferFcn  Denominator=[15 1]
  Out1 : Outport
  wires:
  In1/1 -> Transfer Fcn15/1
  Transfer Fcn16/1 -> Sum6/1
  Transfer Fcn15/1 -> Sum5/1
  Sum5/1 -> Out1/1
  Sum6/1 -> Sum5/2
  Constant/1 -> Transfer Fcn16/1, Sum6/2

== system Main_model/HP Control Systems Battery to Chiller WHR /TF2 ==
  In1 : Inport
  Constant : Constant  Value=ambient_temp
  Sum5 : Sum  Inputs=|++
  Sum6 : Sum  Inputs=|-+
  Transfer Fcn15 : TransferFcn  Denominator=[15 1]
  Transfer Fcn16 : TransferFcn  Denominator=[15 1]
  Out1 : Outport
  wires:
  In1/1 -> Transfer Fcn15/1
  Transfer Fcn16/1 -> Sum6/1
  Transfer Fcn15/1 -> Sum5/1
  Sum5/1 -> Out1/1
  Sum6/1 -> Sum5/2
  Constant/1 -> Transfer Fcn16/1, Sum6/2

== system Main_model/HP Control Systems Battery to Chiller WHR /TF3 ==
  In1 : Inport
  Constant : Constant  Value=ambient_temp
  Sum5 : Sum  Inputs=|++
  Sum6 : Sum  Inputs=|-+
  Transfer Fcn15 : TransferFcn  Denominator=[15 1]
  Transfer Fcn16 : TransferFcn  Denominator=[15 1]
  Out1 : Outport
  wires:
  In1/1 -> Transfer Fcn15/1
  Transfer Fcn16/1 -> Sum6/1
  Transfer Fcn15/1 -> Sum5/1
  Sum5/1 -> Out1/1
  Sum6/1 -> Sum5/2
  Constant/1 -> Transfer Fcn16/1, Sum6/2

== system Main_model/HP Control Systems DT to Battery WHR /HysBat ==
  In1 : Inport
  Relay1 : Relay  OnSwitchValue=T_bat_passive_cool  OffSwitchValue=T_bat_passive_cool-1  OnOutputValue=T_bat_passive_cool*1.1  OffOutputValue=T_bat_passive_cool*.9
  Relay3 : Relay  OnSwitchValue=T_bat_active_cool  OffSwitchValue=T_bat_active_cool-1  OnOutputValue=T_bat_active_cool*1.1  OffOutputValue=T_bat_active_cool*.9
  Switch : Switch  Criteria=u2 > Threshold  Threshold=T_bat_active_cool-5
  Switch1 : Switch  Criteria=u2 > Threshold  Threshold=T_bat_passive_cool-5
  Out1 : Outport
  wires:
  Relay3/1 -> Switch/1
  Switch/1 -> Out1/1
  Relay1/1 -> Switch1/1
  In1/1 -> Relay1/1, Relay3/1, Switch/2, Switch1/2, Switch1/3
  Switch1/1 -> Switch/3

== system Main_model/HP Control Systems DT to Battery WHR /HysDT ==
  In1 : Inport
  Relay2 : Relay  OnSwitchValue=T_DT_passive_cool  OffSwitchValue=T_DT_passive_cool-9  OnOutputValue=T_DT_passive_cool*1.1  OffOutputValue=T_DT_passive_cool*.9
  Relay3 : Relay  OnSwitchValue=T_DT_high  OffSwitchValue=T_DT_high-20  OnOutputValue=T_DT_high*1.1  OffOutputValue=T_DT_high*.9
  Switch : Switch  Criteria=u2 > Threshold  Threshold=T_DT_passive_cool+10
  Out1 : Outport
  wires:
  Relay2/1 -> Switch/3
  Switch/1 -> Out1/1
  Relay3/1 -> Switch/1
  In1/1 -> Relay2/1, Switch/2, Relay3/1

== system Main_model/HP Control Systems DT to Battery WHR /TF ==
  In1 : Inport
  Constant : Constant  Value=T_battery_init
  Sum5 : Sum  Inputs=|++
  Sum6 : Sum  Inputs=|-+
  Transfer Fcn15 : TransferFcn  Denominator=[60 1]
  Transfer Fcn16 : TransferFcn  Denominator=[60 1]
  Out1 : Outport
  wires:
  Constant/1 -> Sum6/2, Transfer Fcn16/1
  Sum6/1 -> Sum5/2
  Sum5/1 -> Out1/1
  Transfer Fcn15/1 -> Sum5/1
  Transfer Fcn16/1 -> Sum6/1
  In1/1 -> Transfer Fcn15/1

== system Main_model/HP Control Systems DT to Battery WHR /TF1 ==
  In1 : Inport
  Constant : Constant  Value=T_cabin_init
  Sum5 : Sum  Inputs=|++
  Sum6 : Sum  Inputs=|-+
  Transfer Fcn15 : TransferFcn  Denominator=[15 1]
  Transfer Fcn16 : TransferFcn  Denominator=[15 1]
  Out1 : Outport
  wires:
  In1/1 -> Transfer Fcn15/1
  Transfer Fcn16/1 -> Sum6/1
  Transfer Fcn15/1 -> Sum5/1
  Sum5/1 -> Out1/1
  Sum6/1 -> Sum5/2
  Constant/1 -> Transfer Fcn16/1, Sum6/2

== system Main_model/HP Control Systems DT to Battery WHR /TF2 ==
  In1 : Inport
  Constant : Constant  Value=ambient_temp
  Sum5 : Sum  Inputs=|++
  Sum6 : Sum  Inputs=|-+
  Transfer Fcn15 : TransferFcn  Denominator=[15 1]
  Transfer Fcn16 : TransferFcn  Denominator=[15 1]
  Out1 : Outport
  wires:
  In1/1 -> Transfer Fcn15/1
  Transfer Fcn16/1 -> Sum6/1
  Transfer Fcn15/1 -> Sum5/1
  Sum5/1 -> Out1/1
  Sum6/1 -> Sum5/2
  Constant/1 -> Transfer Fcn16/1, Sum6/2

== system Main_model/HP Control Systems DT to Battery WHR /TF3 ==
  In1 : Inport
  Constant : Constant  Value=ambient_temp
  Sum5 : Sum  Inputs=|++
  Sum6 : Sum  Inputs=|-+
  Transfer Fcn15 : TransferFcn  Denominator=[15 1]
  Transfer Fcn16 : TransferFcn  Denominator=[15 1]
  Out1 : Outport
  wires:
  In1/1 -> Transfer Fcn15/1
  Transfer Fcn16/1 -> Sum6/1
  Transfer Fcn15/1 -> Sum5/1
  Sum5/1 -> Out1/1
  Sum6/1 -> Sum5/2
  Constant/1 -> Transfer Fcn16/1, Sum6/2

== system Main_model/HP Control Systems Ideal WHR (+ Summer modes) /HysBat ==
  In1 : Inport
  Relay1 : Relay  OnSwitchValue=T_bat_passive_cool  OffSwitchValue=T_bat_passive_cool-1  OnOutputValue=T_bat_passive_cool*1.1  OffOutputValue=T_bat_passive_cool*.9
  Relay3 : Relay  OnSwitchValue=T_bat_active_cool  OffSwitchValue=T_bat_active_cool-1  OnOutputValue=T_bat_active_cool*1.1  OffOutputValue=T_bat_active_cool*.9
  Switch : Switch  Criteria=u2 > Threshold  Threshold=T_bat_active_cool-5
  Switch1 : Switch  Criteria=u2 > Threshold  Threshold=T_bat_passive_cool-5
  Out1 : Outport
  wires:
  Relay3/1 -> Switch/1
  Switch/1 -> Out1/1
  Relay1/1 -> Switch1/1
  In1/1 -> Relay1/1, Relay3/1, Switch/2, Switch1/2, Switch1/3
  Switch1/1 -> Switch/3

== system Main_model/HP Control Systems Ideal WHR (+ Summer modes) /HysDT ==
  In1 : Inport
  Relay2 : Relay  OnSwitchValue=T_DT_passive_cool  OffSwitchValue=T_DT_passive_cool-9  OnOutputValue=T_DT_passive_cool*1.1  OffOutputValue=T_DT_passive_cool*.9
  Relay3 : Relay  OnSwitchValue=T_DT_high  OffSwitchValue=T_DT_high-20  OnOutputValue=T_DT_high*1.1  OffOutputValue=T_DT_high*.9
  Switch : Switch  Criteria=u2 > Threshold  Threshold=T_DT_passive_cool+10
  Out1 : Outport
  wires:
  Relay2/1 -> Switch/3
  Switch/1 -> Out1/1
  Relay3/1 -> Switch/1
  In1/1 -> Relay2/1, Switch/2, Relay3/1

== system Main_model/HP Control Systems Ideal WHR (+ Summer modes) /TF ==
  In1 : Inport
  Constant : Constant  Value=T_battery_init
  Sum5 : Sum  Inputs=|++
  Sum6 : Sum  Inputs=|-+
  Transfer Fcn15 : TransferFcn  Denominator=[60 1]
  Transfer Fcn16 : TransferFcn  Denominator=[60 1]
  Out1 : Outport
  wires:
  Constant/1 -> Sum6/2, Transfer Fcn16/1
  Sum6/1 -> Sum5/2
  Sum5/1 -> Out1/1
  Transfer Fcn15/1 -> Sum5/1
  Transfer Fcn16/1 -> Sum6/1
  In1/1 -> Transfer Fcn15/1

== system Main_model/HP Control Systems Ideal WHR (+ Summer modes) /TF1 ==
  In1 : Inport
  Constant : Constant  Value=T_cabin_init
  Sum5 : Sum  Inputs=|++
  Sum6 : Sum  Inputs=|-+
  Transfer Fcn15 : TransferFcn  Denominator=[15 1]
  Transfer Fcn16 : TransferFcn  Denominator=[15 1]
  Out1 : Outport
  wires:
  In1/1 -> Transfer Fcn15/1
  Transfer Fcn16/1 -> Sum6/1
  Transfer Fcn15/1 -> Sum5/1
  Sum5/1 -> Out1/1
  Sum6/1 -> Sum5/2
  Constant/1 -> Transfer Fcn16/1, Sum6/2

== system Main_model/HP Control Systems Ideal WHR (+ Summer modes) /TF2 ==
  In1 : Inport
  Constant : Constant  Value=ambient_temp
  Sum5 : Sum  Inputs=|++
  Sum6 : Sum  Inputs=|-+
  Transfer Fcn15 : TransferFcn  Denominator=[15 1]
  Transfer Fcn16 : TransferFcn  Denominator=[15 1]
  Out1 : Outport
  wires:
  In1/1 -> Transfer Fcn15/1
  Transfer Fcn16/1 -> Sum6/1
  Transfer Fcn15/1 -> Sum5/1
  Sum5/1 -> Out1/1
  Sum6/1 -> Sum5/2
  Constant/1 -> Transfer Fcn16/1, Sum6/2

== system Main_model/HP Control Systems Ideal WHR (+ Summer modes) /TF3 ==
  In1 : Inport
  Constant : Constant  Value=ambient_temp
  Sum5 : Sum  Inputs=|++
  Sum6 : Sum  Inputs=|-+
  Transfer Fcn15 : TransferFcn  Denominator=[15 1]
  Transfer Fcn16 : TransferFcn  Denominator=[15 1]
  Out1 : Outport
  wires:
  In1/1 -> Transfer Fcn15/1
  Transfer Fcn16/1 -> Sum6/1
  Transfer Fcn15/1 -> Sum5/1
  Sum5/1 -> Out1/1
  Sum6/1 -> Sum5/2
  Constant/1 -> Transfer Fcn16/1, Sum6/2

== system Main_model/HP Control Systems No WHR/HysBat ==
  In1 : Inport
  Relay1 : Relay  OnSwitchValue=T_bat_passive_cool  OffSwitchValue=T_bat_passive_cool-1  OnOutputValue=T_bat_passive_cool*1.1  OffOutputValue=T_bat_passive_cool*.9
  Relay3 : Relay  OnSwitchValue=T_bat_active_cool  OffSwitchValue=T_bat_active_cool-1  OnOutputValue=T_bat_active_cool*1.1  OffOutputValue=T_bat_active_cool*.9
  Switch : Switch  Criteria=u2 > Threshold  Threshold=T_bat_active_cool-5
  Switch1 : Switch  Criteria=u2 > Threshold  Threshold=T_bat_passive_cool-5
  Out1 : Outport
  wires:
  Relay3/1 -> Switch/1
  Switch/1 -> Out1/1
  Relay1/1 -> Switch1/1
  In1/1 -> Relay1/1, Relay3/1, Switch/2, Switch1/2, Switch1/3
  Switch1/1 -> Switch/3

== system Main_model/HP Control Systems No WHR/HysDT ==
  In1 : Inport
  Relay2 : Relay  OnSwitchValue=T_DT_passive_cool  OffSwitchValue=T_DT_passive_cool-9  OnOutputValue=T_DT_passive_cool*1.1  OffOutputValue=T_DT_passive_cool*.9
  Relay3 : Relay  OnSwitchValue=T_DT_high  OffSwitchValue=T_DT_high-20  OnOutputValue=T_DT_high*1.1  OffOutputValue=T_DT_high*.9
  Switch : Switch  Criteria=u2 > Threshold  Threshold=T_DT_passive_cool+10
  Out1 : Outport
  wires:
  Relay2/1 -> Switch/3
  Switch/1 -> Out1/1
  Relay3/1 -> Switch/1
  In1/1 -> Relay2/1, Switch/2, Relay3/1

== system Main_model/HP Control Systems No WHR/TF ==
  In1 : Inport
  Constant : Constant  Value=T_battery_init
  Sum5 : Sum  Inputs=|++
  Sum6 : Sum  Inputs=|-+
  Transfer Fcn15 : TransferFcn  Denominator=[60 1]
  Transfer Fcn16 : TransferFcn  Denominator=[60 1]
  Out1 : Outport
  wires:
  Constant/1 -> Sum6/2, Transfer Fcn16/1
  Sum6/1 -> Sum5/2
  Sum5/1 -> Out1/1
  Transfer Fcn15/1 -> Sum5/1
  Transfer Fcn16/1 -> Sum6/1
  In1/1 -> Transfer Fcn15/1

== system Main_model/HP Control Systems No WHR/TF1 ==
  In1 : Inport
  Constant : Constant  Value=T_cabin_init
  Sum5 : Sum  Inputs=|++
  Sum6 : Sum  Inputs=|-+
  Transfer Fcn15 : TransferFcn  Denominator=[15 1]
  Transfer Fcn16 : TransferFcn  Denominator=[15 1]
  Out1 : Outport
  wires:
  In1/1 -> Transfer Fcn15/1
  Transfer Fcn16/1 -> Sum6/1
  Transfer Fcn15/1 -> Sum5/1
  Sum5/1 -> Out1/1
  Sum6/1 -> Sum5/2
  Constant/1 -> Transfer Fcn16/1, Sum6/2

== system Main_model/HP Control Systems No WHR/TF2 ==
  In1 : Inport
  Constant : Constant  Value=ambient_temp
  Sum5 : Sum  Inputs=|++
  Sum6 : Sum  Inputs=|-+
  Transfer Fcn15 : TransferFcn  Denominator=[15 1]
  Transfer Fcn16 : TransferFcn  Denominator=[15 1]
  Out1 : Outport
  wires:
  In1/1 -> Transfer Fcn15/1
  Transfer Fcn16/1 -> Sum6/1
  Transfer Fcn15/1 -> Sum5/1
  Sum5/1 -> Out1/1
  Sum6/1 -> Sum5/2
  Constant/1 -> Transfer Fcn16/1, Sum6/2

== system Main_model/HP Control Systems No WHR/TF3 ==
  In1 : Inport
  Constant : Constant  Value=ambient_temp
  Sum5 : Sum  Inputs=|++
  Sum6 : Sum  Inputs=|-+
  Transfer Fcn15 : TransferFcn  Denominator=[15 1]
  Transfer Fcn16 : TransferFcn  Denominator=[15 1]
  Out1 : Outport
  wires:
  In1/1 -> Transfer Fcn15/1
  Transfer Fcn16/1 -> Sum6/1
  Transfer Fcn15/1 -> Sum5/1
  Sum5/1 -> Out1/1
  Sum6/1 -> Sum5/2
  Constant/1 -> Transfer Fcn16/1, Sum6/2

== system Main_model/HP Control Systems Only DT to Chiller WHR/HysBat ==
  In1 : Inport
  Relay1 : Relay  OnSwitchValue=T_bat_passive_cool  OffSwitchValue=T_bat_passive_cool-1  OnOutputValue=T_bat_passive_cool*1.1  OffOutputValue=T_bat_passive_cool*.9
  Relay3 : Relay  OnSwitchValue=T_bat_active_cool  OffSwitchValue=T_bat_active_cool-1  OnOutputValue=T_bat_active_cool*1.1  OffOutputValue=T_bat_active_cool*.9
  Switch : Switch  Criteria=u2 > Threshold  Threshold=T_bat_active_cool-5
  Switch1 : Switch  Criteria=u2 > Threshold  Threshold=T_bat_passive_cool-5
  Out1 : Outport
  wires:
  Relay3/1 -> Switch/1
  Switch/1 -> Out1/1
  Relay1/1 -> Switch1/1
  In1/1 -> Relay1/1, Relay3/1, Switch/2, Switch1/2, Switch1/3
  Switch1/1 -> Switch/3

== system Main_model/HP Control Systems Only DT to Chiller WHR/HysDT ==
  In1 : Inport
  Relay2 : Relay  OnSwitchValue=T_DT_passive_cool  OffSwitchValue=T_DT_passive_cool-9  OnOutputValue=T_DT_passive_cool*1.1  OffOutputValue=T_DT_passive_cool*.9
  Relay3 : Relay  OnSwitchValue=T_DT_high  OffSwitchValue=T_DT_high-20  OnOutputValue=T_DT_high*1.1  OffOutputValue=T_DT_high*.9
  Switch : Switch  Criteria=u2 > Threshold  Threshold=T_DT_passive_cool+10
  Out1 : Outport
  wires:
  Relay2/1 -> Switch/3
  Switch/1 -> Out1/1
  Relay3/1 -> Switch/1
  In1/1 -> Relay2/1, Switch/2, Relay3/1

== system Main_model/HP Control Systems Only DT to Chiller WHR/TF ==
  In1 : Inport
  Constant : Constant  Value=T_battery_init
  Sum5 : Sum  Inputs=|++
  Sum6 : Sum  Inputs=|-+
  Transfer Fcn15 : TransferFcn  Denominator=[60 1]
  Transfer Fcn16 : TransferFcn  Denominator=[60 1]
  Out1 : Outport
  wires:
  Constant/1 -> Sum6/2, Transfer Fcn16/1
  Sum6/1 -> Sum5/2
  Sum5/1 -> Out1/1
  Transfer Fcn15/1 -> Sum5/1
  Transfer Fcn16/1 -> Sum6/1
  In1/1 -> Transfer Fcn15/1

== system Main_model/HP Control Systems Only DT to Chiller WHR/TF1 ==
  In1 : Inport
  Constant : Constant  Value=T_cabin_init
  Sum5 : Sum  Inputs=|++
  Sum6 : Sum  Inputs=|-+
  Transfer Fcn15 : TransferFcn  Denominator=[15 1]
  Transfer Fcn16 : TransferFcn  Denominator=[15 1]
  Out1 : Outport
  wires:
  In1/1 -> Transfer Fcn15/1
  Transfer Fcn16/1 -> Sum6/1
  Transfer Fcn15/1 -> Sum5/1
  Sum5/1 -> Out1/1
  Sum6/1 -> Sum5/2
  Constant/1 -> Transfer Fcn16/1, Sum6/2

== system Main_model/HP Control Systems Only DT to Chiller WHR/TF2 ==
  In1 : Inport
  Constant : Constant  Value=ambient_temp
  Sum5 : Sum  Inputs=|++
  Sum6 : Sum  Inputs=|-+
  Transfer Fcn15 : TransferFcn  Denominator=[15 1]
  Transfer Fcn16 : TransferFcn  Denominator=[15 1]
  Out1 : Outport
  wires:
  In1/1 -> Transfer Fcn15/1
  Transfer Fcn16/1 -> Sum6/1
  Transfer Fcn15/1 -> Sum5/1
  Sum5/1 -> Out1/1
  Sum6/1 -> Sum5/2
  Constant/1 -> Transfer Fcn16/1, Sum6/2

== system Main_model/HP Control Systems Only DT to Chiller WHR/TF3 ==
  In1 : Inport
  Constant : Constant  Value=ambient_temp
  Sum5 : Sum  Inputs=|++
  Sum6 : Sum  Inputs=|-+
  Transfer Fcn15 : TransferFcn  Denominator=[15 1]
  Transfer Fcn16 : TransferFcn  Denominator=[15 1]
  Out1 : Outport
  wires:
  In1/1 -> Transfer Fcn15/1
  Transfer Fcn16/1 -> Sum6/1
  Transfer Fcn15/1 -> Sum5/1
  Sum5/1 -> Out1/1
  Sum6/1 -> Sum5/2
  Constant/1 -> Transfer Fcn16/1, Sum6/2
